simulink subsystem "PM100DXR_MC"  (R2023b)
settings: Solver=VariableStepAuto  StartTime=0.0  StopTime=10.0  RelTol=1e-3
settings Model: Creator=diego  LastModifiedBy=nickj

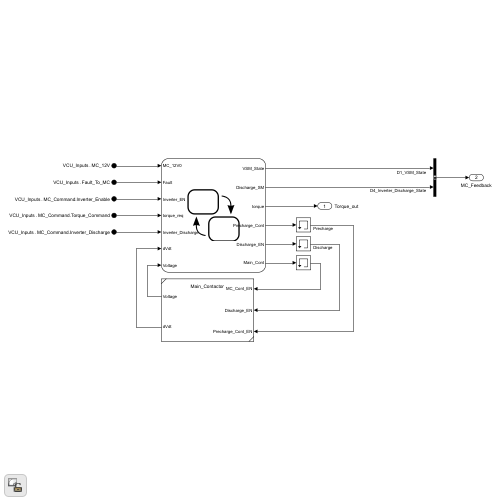
[thumbnail: Simulink's stored preview of the top-level diagram]
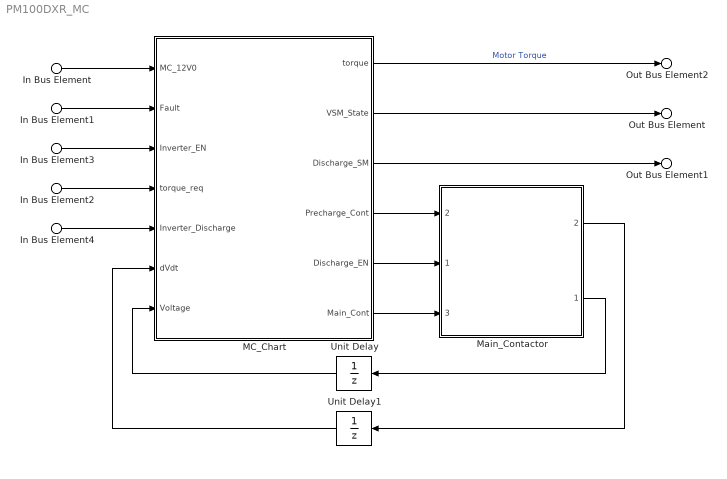
== system PM100DXR_MC ==
  In Bus Element : Inport  PortName=VCU_Inputs  Element=MC_Outputs.MC_12V0
  In Bus Element1 : Inport  PortName=VCU_Inputs  Element=MC_Outputs.Fault_To_MC
  In Bus Element3 : Inport  PortName=VCU_Inputs  Element=VCU_Outputs.Inverter_Enable
  In Bus Element2 : Inport  PortName=VCU_Inputs  Element=VCU_Outputs.Torque_Command
  In Bus Element4 : Inport  PortName=VCU_Inputs  Element=VCU_Outputs.Inverter_Discharge
  MC_Chart : Stateflow chart  TreatAsAtomicUnit=on
      settings: PortSchema="{\"entries\":[{\"content\":{\"sides\":[{\"content\":{\"connectorIds\":[\"In3\",\"In1\",\"In2\",\"In6\",\"In4\",\"In7\",\"In5\"]},\"type\":\"ConnectorPlacement.EquallySpacedRectSide\",\"uuid\":\"03599179-c40e-45c0-8f83-03707e7643a9\"},{\"content\":{\"connectorIds\":[\"Out6\",\"Out1\",\"Out2\",\"Out3\",\"Out4\",\"Out5\"],\"side\":\"RIGHT\"},\"type\":\"ConnectorPlacement.EquallySpacedRectSide\",\"uuid\":\"77c27c81-6b7f-49bb-b8ad-65b312eda7e2\"},{\"content\":{\"side\":\"TOP\"},\"type\":\"ConnectorPlacement.EquallySpacedRectSide\",\"uuid\":\"12a0a04d-7874-431f-b4d8-e9223037e866\"}]},\"type\":\"ConnectorPlacement.EquallySpacedConnector\",\"uuid\":\"58e614a8-4325-4fa7-852b-761998465240\"}],\"packageUris\":[\"http://schema.mathworks.com/mf0/Connector/R2020b\"],\"version\":\"1.0\"}"
  Main_Contactor : Subsystem  ReferencedSubsystem=Main_Contactor
      settings: PortSchema="{\"entries\":[{\"content\":{\"sides\":[{\"content\":{\"connectorIds\":[\"In3\",\"In1\",\"In2\"]},\"type\":\"ConnectorPlacement.EquallySpacedRectSide\",\"uuid\":\"c4a26b2a-75b7-46e9-83ad-f08a209eb654\"},{\"content\":{\"connectorIds\":[\"Out1\",\"Out2\"],\"side\":\"RIGHT\"},\"type\":\"ConnectorPlacement.EquallySpacedRectSide\",\"uuid\":\"e0e23db8-3606-4757-a6fd-db7c1d3e8c5a\"},{\"content\":{\"side\":\"TOP\"},\"type\":\"ConnectorPlacement.EquallySpacedRectSide\",\"uuid\":\"0a967cd1-2252-4813-adc7-d3e8433b462a\"}]},\"type\":\"ConnectorPlacement.EquallySpacedConnector\",\"uuid\":\"d4c2dd3c-9ab6-4575-a91c-d1aa35d96284\"}],\"packageUris\":[\"http://schema.mathworks.com/mf0/Connector/R2020b\"],\"version\":\"1.0\"}"
  Unit Delay : UnitDelay  SampleTime=-1  HasFrameUpgradeWarning=on
  Unit Delay1 : UnitDelay  SampleTime=-1  HasFrameUpgradeWarning=on
  Out Bus Element2 : Outport  PortName=Motor_Outputs  Element=Torque
  Out Bus Element : Outport  Port=2  PortName=MC_Feedback  Element=D1_VSM_State
  Out Bus Element1 : Outport  Port=2  PortName=MC_Feedback  Element=D4_Inverter_Discharge_State
  wires:
  MC_Chart/3(Precharge_Cont) -> Main_Contactor/2
  In Bus Element1/1 -> MC_Chart/1(Fault)
  In Bus Element/1 -> MC_Chart/3(MC_12V0)
  In Bus Element3/1 -> MC_Chart/2(Inverter_EN)
  MC_Chart/4(Discharge_EN) -> Main_Contactor/1
  MC_Chart/6(torque) -> Out Bus Element2/1  "Motor Torque"
  MC_Chart/5(Main_Cont) -> Main_Contactor/3
  In Bus Element4/1 -> MC_Chart/4(Inverter_Discharge)
  In Bus Element2/1 -> MC_Chart/6(torque_req)
  Main_Contactor/1 -> Unit Delay/1
  Unit Delay/1 -> MC_Chart/5(Voltage)
  Main_Contactor/2 -> Unit Delay1/1
  Unit Delay1/1 -> MC_Chart/7(dVdt)
  MC_Chart/1(VSM_State) -> Out Bus Element/1
  MC_Chart/2(Discharge_SM) -> Out Bus Element1/1

== stateflow chart PM100DXR_MC/MC_Chart ==
  state Motor_Controller
    state Power_ON
      entry:
      VSM_State = MC_VSM_State.Start;
      Discharge_SM = MC_DC_State.Disabled;
    state Precharge
      entry:
      VSM_State = MC_VSM_State.PC_Init;
      Discharged = false;
      state Precharge2
        during:
        VSM_State = MC_VSM_State.PC_Finish;
        dV = dVdt;
      state Precharge3
        entry:
        VSM_State = MC_VSM_State.Wait;
        Precharge_Cont = false;
        Main_Cont = true;
      state Precharge1
        during:
        VSM_State = MC_VSM_State.PC_Active;
        dV = 1000;
        Precharge_Cont = true;
      (default) -> Precharge1
      Precharge1 -> Precharge2 : [dV ~= dVdt]
      Precharge2 -> Precharge3 : [dV<56]
    state Fault
      entry:
      VSM_State = MC_VSM_State.Fault;
    state Running
      entry:
      VSM_State = MC_VSM_State.Motor_Running;
      during:
      torque = torque_req;
      exit:
      torque = 0;
    state Ready
      entry:
      VSM_State = MC_VSM_State.Ready;
    state Shutdown
      entry:
      VSM_State = MC_VSM_State.Shutdown;
      Discharge_EN = false;
      Discharged = true;
    state Discharge
      entry:
      VSM_State = MC_VSM_State.Shutdown;
      Main_Cont = false;
      state Discharge1
        entry:
        Discharge_SM = MC_DC_State.Enabled;
        Discharge_EN = true;
      state Discharge2
        entry:
        Discharge_SM = MC_DC_State.Speed_Check;
      state Discharge4
        entry:
        Discharge_SM = MC_DC_State.Complete;
      state Discharge3
        entry:
        Discharge_SM = MC_DC_State.Active;
      (default) -> Discharge1
      Discharge1 -> Discharge2
      Discharge2 -> Discharge3 : [RPM < 75]
      Discharge3 -> Discharge4 : [ Voltage < 30]
    (default) -> Power_ON
    Shutdown -> Power_ON : [MC_12V0 == false]
    Power_ON -> Precharge : [MC_12V0 == true]
    Precharge3 -> Ready
    Motor_Controller -> Fault [order 2] : [Fault == true  && Discharge_EN ~= false && MC_12V0 == true]
    Ready -> Running : [Inverter_EN == true && torque_req == 0]
    Running -> Ready : [Inverter_EN == false]
    Fault -> Discharge : [MC_12V0 == false]
    Discharge -> Shutdown : [Discharge_SM == MC_DC_State.Complete]
    Motor_Controller -> Discharge [order 1] : [Inverter_Discharge == true && VSM_State ~= MC_VSM_State.Shutdown && Discharged == false]
  (default) -> Motor_Controller
  data: Fault input; VSM_State output =MC_VSM_State.Start; Inverter_EN input; Discharge_SM output =MC_DC_State.Enabled; RPM local =0; MC_12V0 input; Inverter_Discharge input; Precharge_Cont output; Voltage input =0; Discharge_EN output =false; Main_Cont output =false; torque_req input; torque output; dVdt input; dV local =1000; Discharged local =true
